simulink model "wiadro"  (R2020b)
settings: Solver=VariableStepAuto  StartTime=0.0  StopTime=720  RelTol=1e-3
settings Model: Creator=matis  LastModifiedBy=matis

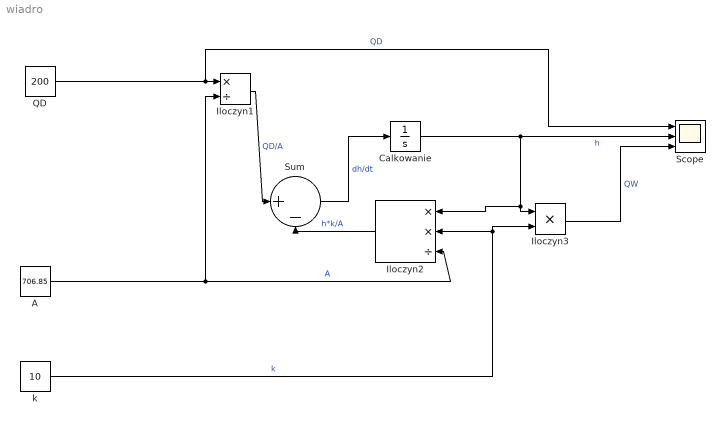
== system wiadro ==
  A : Constant  Value=706.85
  Calkowanie : Integrator  InitialCondition=10
  Iloczyn1 : Product  Inputs=*/
  Iloczyn2 : Product  Inputs=**/
  Iloczyn3 : Product
  QD : Constant  Value=200
  Scope : Scope  NumInputPorts=3
  Sum : Sum  Inputs=|+-
  k : Constant  Value=10
  wires:
  QD/1 -> Scope/1, Iloczyn1/1  "QD"
  Iloczyn1/1 -> Sum/1  "QD/A"
  A/1 -> Iloczyn1/2, Iloczyn2/3  "A"
  Iloczyn2/1 -> Sum/2  "h*k/A"
  Sum/1 -> Calkowanie/1  "dh/dt"
  Calkowanie/1 -> Iloczyn2/1, Iloczyn3/1, Scope/2  "h"
  Iloczyn3/1 -> Scope/3  "QW"
  k/1 -> Iloczyn3/2, Iloczyn2/2  "k"
